simulink library "TYPEBP_MASTER"  (Simulink 8.6)
settings: Solver=ode45  StartTime=0.0  StopTime=10.0  RelTol=1e-3
undefined symbols (not defined in the file): TYPEC, TYPEC_MASTER
libraries: cdsEpicsOut x38, cdsFilt x34, cdsFiltCtrl x24, STATE_BIO_MASTER x18, cdsTP x16, cdsEpicsBinIn x9, VIS_LIB x8, cdsEpicsIn x8, cdsMuxMatrix x5, SIXOSEM_F_STAGE_MASTER x4, cdsEpicsStringIn x3, cdsDacKill x3
(part 3 of 8)

== system TYPEBP_MASTER/TYPEBPMASTER_TEST/TEST ==
  In1 : Inport
  In4 : Inport  Port=2
  In7 : Inport  Port=3
  In10 : Inport  Port=4
  CH1 : cdsFiltCtrl/IIR FM with control  Tag=cdsFiltCtrl  Description=|
      | cdsFiltCntrl is the standard IIR filter module (exactly the same as cdsFilt) but with added control data output 'Ctrl'. Filter module digital signal output appears on the first output, which is called 'Val'. 'Ctrl' output has a bit pattern encoding the state of filter's on/off switches (FM1 through FM10). The bit values are:
      |                                                                                                                                                                                                                                                                                                                                       
      | module 	hex	dec                                                                                                                                                                                                                                                                                                                       
      | -----------------------                                                                                                                                                                                                                                                                                                               
      | FM1	0x20                    32                                                                                                                                                                                                                                                                                                        
      | FM2	0x80                     128                                                                                                                                                                                                                                                                                                      
      | FM3	0x200                   512                                                                                                                                                                                                                                                                                                       
      | FM4	0x800                   2048                                                                                                                                                                                                                                                                                                      
      | FM5	0x2000                 8192                                                                                                                                                                                                                                                                                                       
      | FM6	0x8000                 32768                                                                                                                                                                                                                                                                                                      
      | FM7	0x20000                131072                                                                                                                                                                                                                                                                                                     
      | FM8	0x80000                 524288                                                                                                                                                                                                                                                                                                    
      | FM9	0x200000               2097152                                                                                                                                                                                                                                                                                                    
      | FM10	0x800000               8388608                                                                                                                                                                                                                                                                                                   
      |                                                                                                                                                                                                                                                                                                                                       
      | This bit data can be used to drive some other switches or it can be output using a binary I/O module.
      settings: AttributesFormatString=%<Tag>
  CH2 : cdsFiltCtrl/IIR FM with control  Tag=cdsFiltCtrl  Description=|
      | cdsFiltCntrl is the standard IIR filter module (exactly the same as cdsFilt) but with added control data output 'Ctrl'. Filter module digital signal output appears on the first output, which is called 'Val'. 'Ctrl' output has a bit pattern encoding the state of filter's on/off switches (FM1 through FM10). The bit values are:
      |                                                                                                                                                                                                                                                                                                                                       
      | module 	hex	dec                                                                                                                                                                                                                                                                                                                       
      | -----------------------                                                                                                                                                                                                                                                                                                               
      | FM1	0x20                    32                                                                                                                                                                                                                                                                                                        
      | FM2	0x80                     128                                                                                                                                                                                                                                                                                                      
      | FM3	0x200                   512                                                                                                                                                                                                                                                                                                       
      | FM4	0x800                   2048                                                                                                                                                                                                                                                                                                      
      | FM5	0x2000                 8192                                                                                                                                                                                                                                                                                                       
      | FM6	0x8000                 32768                                                                                                                                                                                                                                                                                                      
      | FM7	0x20000                131072                                                                                                                                                                                                                                                                                                     
      | FM8	0x80000                 524288                                                                                                                                                                                                                                                                                                    
      | FM9	0x200000               2097152                                                                                                                                                                                                                                                                                                    
      | FM10	0x800000               8388608                                                                                                                                                                                                                                                                                                   
      |                                                                                                                                                                                                                                                                                                                                       
      | This bit data can be used to drive some other switches or it can be output using a binary I/O module.
      settings: AttributesFormatString=%<Tag>
  CH3 : cdsFiltCtrl/IIR FM with control  Tag=cdsFiltCtrl  Description=|
      | cdsFiltCntrl is the standard IIR filter module (exactly the same as cdsFilt) but with added control data output 'Ctrl'. Filter module digital signal output appears on the first output, which is called 'Val'. 'Ctrl' output has a bit pattern encoding the state of filter's on/off switches (FM1 through FM10). The bit values are:
      |                                                                                                                                                                                                                                                                                                                                       
      | module 	hex	dec                                                                                                                                                                                                                                                                                                                       
      | -----------------------                                                                                                                                                                                                                                                                                                               
      | FM1	0x20                    32                                                                                                                                                                                                                                                                                                        
      | FM2	0x80                     128                                                                                                                                                                                                                                                                                                      
      | FM3	0x200                   512                                                                                                                                                                                                                                                                                                       
      | FM4	0x800                   2048                                                                                                                                                                                                                                                                                                      
      | FM5	0x2000                 8192                                                                                                                                                                                                                                                                                                       
      | FM6	0x8000                 32768                                                                                                                                                                                                                                                                                                      
      | FM7	0x20000                131072                                                                                                                                                                                                                                                                                                     
      | FM8	0x80000                 524288                                                                                                                                                                                                                                                                                                    
      | FM9	0x200000               2097152                                                                                                                                                                                                                                                                                                    
      | FM10	0x800000               8388608                                                                                                                                                                                                                                                                                                   
      |                                                                                                                                                                                                                                                                                                                                       
      | This bit data can be used to drive some other switches or it can be output using a binary I/O module.
      settings: AttributesFormatString=%<Tag>
  CH4 : cdsFiltCtrl/IIR FM with control  Tag=cdsFiltCtrl  Description=|
      | cdsFiltCntrl is the standard IIR filter module (exactly the same as cdsFilt) but with added control data output 'Ctrl'. Filter module digital signal output appears on the first output, which is called 'Val'. 'Ctrl' output has a bit pattern encoding the state of filter's on/off switches (FM1 through FM10). The bit values are:
      |                                                                                                                                                                                                                                                                                                                                       
      | module 	hex	dec                                                                                                                                                                                                                                                                                                                       
      | -----------------------                                                                                                                                                                                                                                                                                                               
      | FM1	0x20                    32                                                                                                                                                                                                                                                                                                        
      | FM2	0x80                     128                                                                                                                                                                                                                                                                                                      
      | FM3	0x200                   512                                                                                                                                                                                                                                                                                                       
      | FM4	0x800                   2048                                                                                                                                                                                                                                                                                                      
      | FM5	0x2000                 8192                                                                                                                                                                                                                                                                                                       
      | FM6	0x8000                 32768                                                                                                                                                                                                                                                                                                      
      | FM7	0x20000                131072                                                                                                                                                                                                                                                                                                     
      | FM8	0x80000                 524288                                                                                                                                                                                                                                                                                                    
      | FM9	0x200000               2097152                                                                                                                                                                                                                                                                                                    
      | FM10	0x800000               8388608                                                                                                                                                                                                                                                                                                   
      |                                                                                                                                                                                                                                                                                                                                       
      | This bit data can be used to drive some other switches or it can be output using a binary I/O module.
      settings: AttributesFormatString=%<Tag>
  Ground{1..6,19,22} (8 alike) : Ground
  Terminator{1..5,16..18} (8 alike) : Terminator
  wires:
  CH4/2 -> Terminator1/1
  Ground5/1 -> CH4/3
  Ground6/1 -> CH4/2
  Ground3/1 -> CH3/3
  Ground4/1 -> CH3/2
  Ground1/1 -> CH2/3
  Ground2/1 -> CH2/2
  CH3/2 -> Terminator18/1
  CH2/2 -> Terminator17/1
  CH1/2 -> Terminator16/1
  Ground19/1 -> CH1/3
  Ground22/1 -> CH1/2
  In10/1 -> CH4/1
  In7/1 -> CH3/1
  In1/1 -> CH1/1
  CH2/1 -> Terminator4/1
  In4/1 -> CH2/1
  CH4/1 -> Terminator2/1
  CH3/1 -> Terminator3/1
  CH1/1 -> Terminator5/1

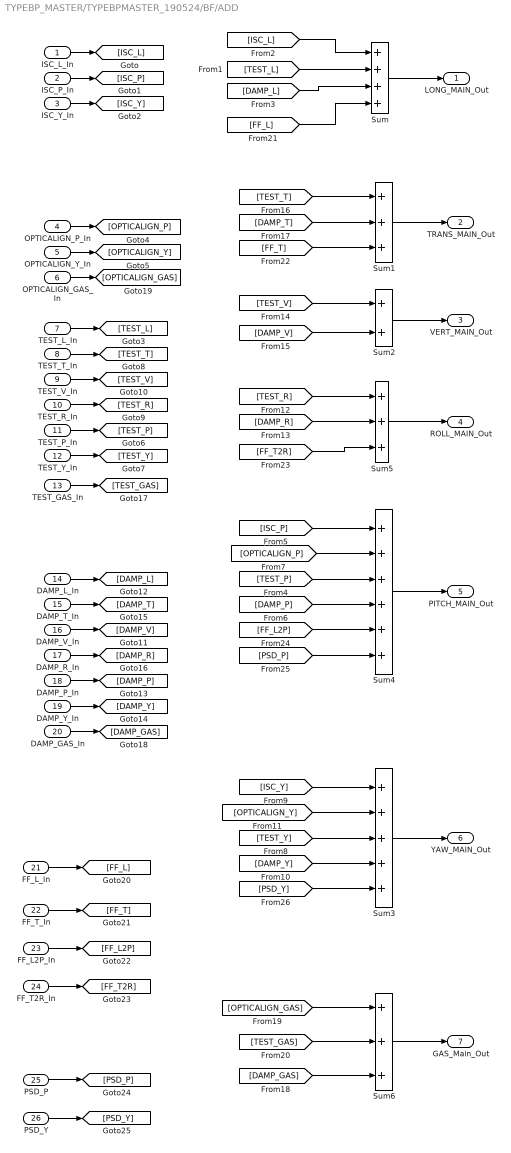
== system TYPEBP_MASTER/TYPEBPMASTER_190524/BF/ADD ==
  ISC_L_In : Inport
  ISC_P_In : Inport  Port=2
  ISC_Y_In : Inport  Port=3
  OPTICALIGN_P_In : Inport  Port=4
  OPTICALIGN_Y_In : Inport  Port=5
  OPTICALIGN_GAS_In : Inport  Port=6
  TEST_L_In : Inport  Port=7
  TEST_T_In : Inport  Port=8
  TEST_V_In : Inport  Port=9
  TEST_R_In : Inport  Port=10
  TEST_P_In : Inport  Port=11
  TEST_Y_In : Inport  Port=12
  TEST_GAS_In : Inport  Port=13
  DAMP_L_In : Inport  Port=14
  DAMP_T_In : Inport  Port=15
  DAMP_V_In : Inport  Port=16
  DAMP_R_In : Inport  Port=17
  DAMP_P_In : Inport  Port=18
  DAMP_Y_In : Inport  Port=19
  DAMP_GAS_In : Inport  Port=20
  FF_L_In : Inport  Port=21
  FF_T_In : Inport  Port=22
  FF_L2P_In : Inport  Port=23
  FF_T2R_In : Inport  Port=24
  PSD_P : Inport  Port=25
  PSD_Y : Inport  Port=26
  Sum : Sum  Inputs=++++
  Sum1 : Sum  Inputs=+++
  Sum2 : Sum
  Sum3 : Sum  Inputs=+++++
  Sum4 : Sum  Inputs=++++++
  Sum5 : Sum  Inputs=+++
  Sum6 : Sum  Inputs=+++
  LONG_MAIN_Out : Outport
  TRANS_MAIN_Out : Outport  Port=2
  VERT_MAIN_Out : Outport  Port=3
  ROLL_MAIN_Out : Outport  Port=4
  PITCH_MAIN_Out : Outport  Port=5
  YAW_MAIN_Out : Outport  Port=6
  GAS_Main_Out : Outport  Port=7
  wires:
  [PSD_Y] -> Sum3/5
  [PSD_P] -> Sum4/6
  PSD_P/1 -> [PSD_P]
  PSD_Y/1 -> [PSD_Y]
  [DAMP_V] -> Sum2/2
  [TEST_V] -> Sum2/1
  [DAMP_T] -> Sum1/2
  [TEST_T] -> Sum1/1
  [DAMP_R] -> Sum5/2
  [TEST_R] -> Sum5/1
  [DAMP_Y] -> Sum3/4
  [TEST_Y] -> Sum3/3
  [OPTICALIGN_Y] -> Sum3/2
  [ISC_Y] -> Sum3/1
  [DAMP_P] -> Sum4/4
  [TEST_P] -> Sum4/3
  [OPTICALIGN_P] -> Sum4/2
  [ISC_P] -> Sum4/1
  ISC_Y_In/1 -> [ISC_Y]
  ISC_P_In/1 -> [ISC_P]
  ISC_L_In/1 -> [ISC_L]
  OPTICALIGN_Y_In/1 -> [OPTICALIGN_Y]
  OPTICALIGN_P_In/1 -> [OPTICALIGN_P]
  Sum1/1 -> TRANS_MAIN_Out/1
  Sum2/1 -> VERT_MAIN_Out/1
  Sum5/1 -> ROLL_MAIN_Out/1
  [DAMP_L] -> Sum/3
  [TEST_L] -> Sum/2
  [ISC_L] -> Sum/1
  Sum/1 -> LONG_MAIN_Out/1
  Sum3/1 -> YAW_MAIN_Out/1
  Sum4/1 -> PITCH_MAIN_Out/1
  Sum6/1 -> GAS_Main_Out/1
  OPTICALIGN_GAS_In/1 -> [OPTICALIGN_GAS]
  TEST_L_In/1 -> [TEST_L]
  TEST_T_In/1 -> [TEST_T]
  TEST_V_In/1 -> [TEST_V]
  TEST_R_In/1 -> [TEST_R]
  TEST_P_In/1 -> [TEST_P]
  TEST_Y_In/1 -> [TEST_Y]
  TEST_GAS_In/1 -> [TEST_GAS]
  DAMP_L_In/1 -> [DAMP_L]
  DAMP_T_In/1 -> [DAMP_T]
  DAMP_V_In/1 -> [DAMP_V]
  DAMP_R_In/1 -> [DAMP_R]
  DAMP_P_In/1 -> [DAMP_P]
  DAMP_Y_In/1 -> [DAMP_Y]
  DAMP_GAS_In/1 -> [DAMP_GAS]
  [OPTICALIGN_GAS] -> Sum6/1
  [TEST_GAS] -> Sum6/2
  [DAMP_GAS] -> Sum6/3
  FF_L_In/1 -> [FF_L]
  FF_T_In/1 -> [FF_T]
  [FF_L] -> Sum/4
  [FF_T] -> Sum1/3
  FF_L2P_In/1 -> [FF_L2P]
  [FF_T2R] -> Sum5/3
  [FF_L2P] -> Sum4/5
  FF_T2R_In/1 -> [FF_T2R]
